simulink model "s_waage5"  (Simulink 4.00)
settings: Solver=ode15s  SolverMode=SingleTasking  StartTime=0.0  StopTime=0.25  FixedStep=1e-4  MaxStep=1e-4  RelTol=1e-3  AbsTol=1e-6
values from neighbouring files (symbols this model uses):
  D = my_sys1.d    [ncd_estim1.m]    (also in ncd_estim_1.mat = 0; ncd_kalm1.m; ncd_kalm2.m; ncd_kalm_1.mat = 0)
  g = 9.8    [ident21.mat]    (also in torce11.m = 9.81; torcell.mat = 9.81; waag11.m = 9.81; waag11.mat = 9.81)
  kg = 5    [waag11.m]    (also in waag11.mat; waage2.m; waage3.m)
  ks = 200    [waag11.m]    (also in waag11.mat; waage2.m; waage3.m = 300)
  L = place(A, B, p)'    [ncd_estim1.m]    (also in ncd_estim_1.mat = [29.04 93.6748 304.13176 464.47352 317.56952 149.5392]; ncd_kalm_2.mat = [29.04 93.6748 304.13176 464.47352 317.56952 149.5392]; torce11.m = axis; torcell.mat = [0 100 0 3])
  mw = 0.1    [waag11.m]    (also in waag11.mat; waage2.m; waage3.m = 0.5)
  mx = 5    [waag11.m]    (also in waag11.mat; waage2.m; waage3.m)
  R = 1    [ncd_estim1.m]    (also in ncd_estim_1.mat; ncd_kalm1.m; ncd_kalm2.m; ncd_kalm_1.mat)
  r = 0.0003    [ident21.mat]    (also in waag11.m = 100; waag11.mat = 100; waage2.m = 100; waage3.m = 100)
  Ts = 1e-3    (= 0.001)    [waage3.m]
undefined symbols (not defined in the file or in its folder): dend, numd
settings Model: LastModifiedBy=Administrator  SaveTime=off  SaveOutput=off  LimitDataPoints=off  BlockReductionOpt=off

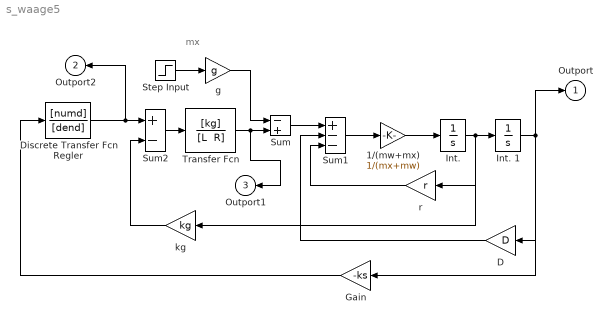
== system s_waage5 ==
  note: mx
  1/(mw+mx) : Gain  Gain=1/(mx+mw)  Multiplication=Element-wise(K.*u)  SaturateOnIntegerOverflow=on
  D : Gain  Orientation=left  Gain=D  Multiplication=Element-wise(K.*u)  SaturateOnIntegerOverflow=on
  Discrete Transfer Fcn Regler : DiscreteTransferFcn  Numerator=[numd]  Denominator=[dend]  SampleTime=Ts  Realization=auto
  Gain : Gain  Orientation=left  Gain=-ks  Multiplication=Element-wise(K.*u)  SaturateOnIntegerOverflow=on
  Int. : Integrator  ExternalReset=none  InitialConditionSource=internal  InitialCondition=0  LimitOutput=off  UpperSaturationLimit=inf  LowerSaturationLimit=-inf  ShowSaturationPort=off  ShowStatePort=off  AbsoluteTolerance=auto
  Int. 1 : Integrator  ExternalReset=none  InitialConditionSource=internal  InitialCondition=0  LimitOutput=off  UpperSaturationLimit=inf  LowerSaturationLimit=-inf  ShowSaturationPort=off  ShowStatePort=off  AbsoluteTolerance=auto
  Step Input : Step  Time=0  Before=0  After=mx  SampleTime=-1
  Sum : Sum  Inputs=-+  SaturateOnIntegerOverflow=on
  Sum1 : Sum  Inputs=+--  SaturateOnIntegerOverflow=on
  Sum2 : Sum  Inputs=+-  SaturateOnIntegerOverflow=on
  Transfer Fcn : TransferFcn  Numerator=[kg]  Denominator="[L  R]"  Realization=auto  AbsoluteTolerance=auto
  g : Gain  Gain=g  Multiplication=Element-wise(K.*u)  SaturateOnIntegerOverflow=on
  kg : Gain  Orientation=left  Gain=kg  Multiplication=Element-wise(K.*u)  SaturateOnIntegerOverflow=on
  r : Gain  Orientation=left  Gain=r  Multiplication=Element-wise(K.*u)  SaturateOnIntegerOverflow=on
  Outport : Outport  Port=1  InitialOutput=0
  Outport2 : Outport  Orientation=left  Port=2  InitialOutput=0
  Outport1 : Outport  Orientation=left  Port=3  InitialOutput=0
  wires:
  Transfer Fcn/1 -> Outport1/1, Sum/2
  kg/1 -> Sum2/2
  Discrete Transfer Fcn Regler/1 -> Sum2/1, Outport2/1
  Gain/1 -> Discrete Transfer Fcn Regler/1
  Int. 1/1 -> Gain/1, Outport/1, D/1
  Sum2/1 -> Transfer Fcn/1
  r/1 -> Sum1/3
  Int./1 -> kg/1, r/1, Int. 1/1
  D/1 -> Sum1/2
  1/(mw+mx)/1 -> Int./1
  Sum1/1 -> 1/(mw+mx)/1
  Sum/1 -> Sum1/1
  g/1 -> Sum/1
  Step Input/1 -> g/1
